simulink model "Problem9_BLDC_Motor"  (R2020b)
settings: Solver=ode45  StartTime=0.0  StopTime=5  MaxStep=0.001  RelTol=1e-5
libraries: fl_lib x23, fl_ps_legacy_lib x15, nesl_utility x7, ee_lib x1
settings Model: Creator=vigne  LastModifiedBy=vigne

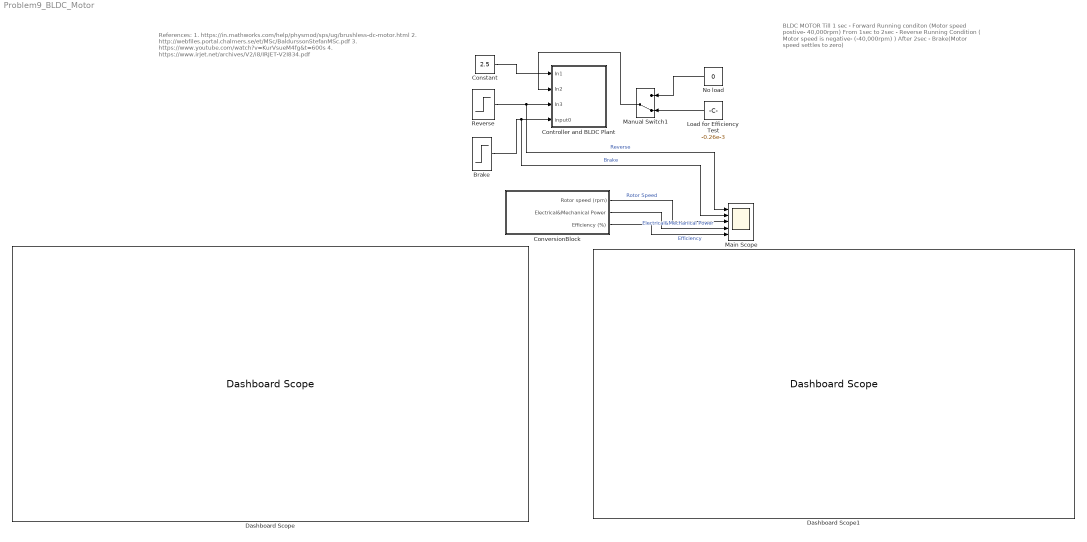
== system Problem9_BLDC_Motor ==
  note: BLDC MOTOR
      |
      | Till 1 sec - Forward Running conditon (Motor speed postive- 40,000rpm)
      |
      | From 1sec to 2sec - Reverse Running Condition ( Motor speed is negative- (-40,000rpm) )
      |
      | After 2sec - Brake(Motor speed settles to zero)
  note: References:
      |
      | 1. https://in.mathworks.com/help/physmod/sps/ug/brushless-dc-motor.html
      | 2. http://webfiles.portal.chalmers.se/et/MSc/BaldurssonStefanMSc.pdf
      | 3. https://www.youtube.com/watch?v=KurVsueM4fg&t=600s
      | 4. https://www.irjet.net/archives/V2/i8/IRJET-V2I834.pdf
  Brake : Step  Time=2  After=5  SampleTime=0
  Constant : Constant  Value=2.5
  Controller and BLDC Plant : Subsystem
  ConversionBlock : Subsystem
  Dashboard Scope : DashboardScope
  Dashboard Scope1 : DashboardScope
  Load for Efficiency Test : Constant  Value=-0.26e-3
  Main Scope : Scope  NumInputPorts=5
  Manual Switch1 : ManualSwitch  CurrentSetting=0
  No load : Constant  Value=0
  Reverse : Step  After=5  SampleTime=0
  wires:
  Load for Efficiency Test/1 -> Manual Switch1/2
  No load/1 -> Manual Switch1/1
  ConversionBlock/1(Rotor speed (rpm)) -> Main Scope/3  "Rotor Speed"
  ConversionBlock/2(Electrical&Mechanical Power) -> Main Scope/4  "Electrical&Mechanical Power"
  ConversionBlock/3(Efficiency (%)) -> Main Scope/5  "Efficiency"
  Constant/1 -> Controller and BLDC Plant/1(In1)
  Manual Switch1/1 -> Controller and BLDC Plant/2(In2)
  Reverse/1 -> Main Scope/1, Controller and BLDC Plant/3(In3)  "Reverse"
  Brake/1 -> Main Scope/2, Controller and BLDC Plant/4(input0)  "Brake"

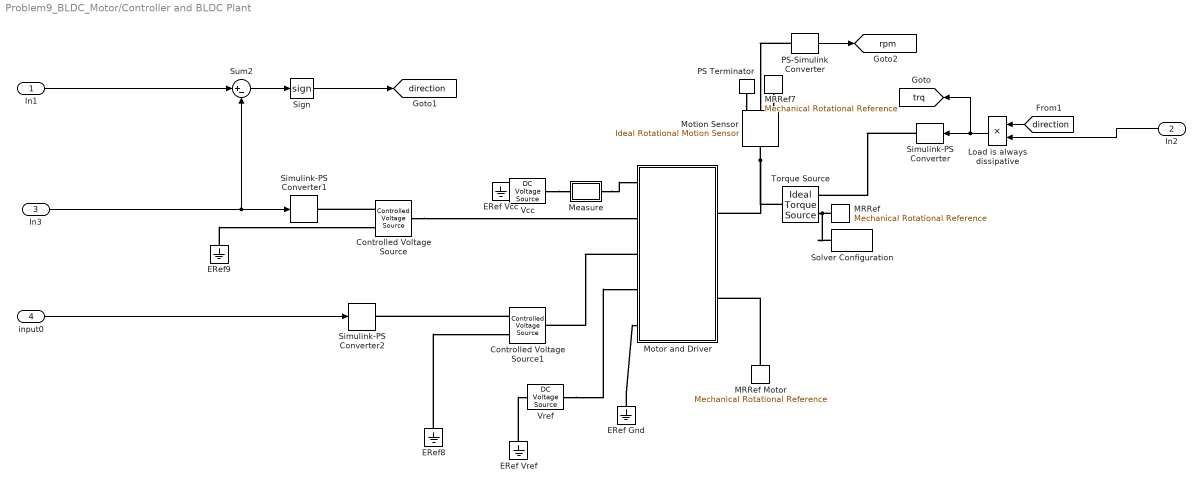
== system Problem9_BLDC_Motor/Controller and BLDC Plant ==
  In1 : Inport
  In2 : Inport  Port=2
  In3 : Inport  Port=3
  input0 : Inport  Port=4
  Controlled Voltage Source : fl_lib/Electrical/Electrical Sources/Controlled Voltage Source
      settings: SourceProductName=Foundation Library
  Controlled Voltage Source1 : fl_lib/Electrical/Electrical Sources/Controlled Voltage Source
      settings: SourceProductName=Foundation Library
  ERef Vcc : fl_lib/Electrical/Electrical Elements/Electrical Reference
      settings: SourceProductName=Foundation Library
  ERef Vref : fl_lib/Electrical/Electrical Elements/Electrical Reference
      settings: SourceProductName=Foundation Library
  ERef Gnd : fl_lib/Electrical/Electrical Elements/Electrical Reference
      settings: SourceProductName=Foundation Library
  ERef8 : fl_lib/Electrical/Electrical Elements/Electrical Reference
      settings: SourceProductName=Foundation Library
  ERef9 : fl_lib/Electrical/Electrical Elements/Electrical Reference
      settings: SourceProductName=Foundation Library
  Load is always dissipative : Product  InputSameDT=on  SaturateOnIntegerOverflow=on  OutDataTypeStr=Inherit: Same as first input
  MRRef : fl_lib/Mechanical/Rotational Elements/Mechanical Rotational Reference
      settings: SourceProductName=Foundation Library
  MRRef Motor : fl_lib/Mechanical/Rotational Elements/Mechanical Rotational Reference
      settings: SourceProductName=Foundation Library
  MRRef7 : fl_lib/Mechanical/Rotational Elements/Mechanical Rotational Reference
      settings: SourceProductName=Foundation Library
  Measure : Subsystem
      mask Display: disp('S');
  Motion Sensor : fl_lib/Mechanical/Mechanical Sensors/Ideal Rotational Motion Sensor  wrap_angle=simscape.enum.onoff.off  offset=0 rad
      settings: SourceProductName=Foundation Library
  Motor and Driver : Subsystem  Tag=PublishSubsystem  mask(Servomotor & Driver){Vcc=12, I0=44e-3, T_i=0.5e-3, eta=41, rpm_eta=40000, trq_eta=0.26e-3, trq_stall=0.44e-3, Kp=0.0000001, Ki=0.000004, Vref_max=5, rpm_max=100000, J=5e-10, rpm0=0}
      mask prompts: Vcc "Nominal voltage (V)"; I0 "No-load DC current to driver (A)"; T_i "Current loop time constant (s)"; eta "Efficiency (%)"; rpm_eta "Speed at which efficiency measured (rpm)"; trq_eta "Torque at which efficiency measured  (Nm)"; trq_stall "Stall torque (Nm)"; Kp "Proportional gain"; Ki "Integral gain"; Vref_max "Maximum reference voltage (V)"; rpm_max "Speed at maximum reference voltage (rpm)"; J "Rotor inerita (kg*m^2)"; rpm0 "Rotor initial speed (rpm)"
      mask help: Implements an abstracted model of a servomotor and driver configured for closed-loop speed control.
      mask DialogControl ParameterTabVar0 Prompt: Electrical
      mask DialogControl ParameterTabVar01 Prompt: Efficiency
      mask DialogControl ParameterTabVar012 Prompt: Mechanical
      mask DialogControl ParameterTabVar0123 Prompt: Controller
  PS Terminator : fl_lib/Physical Signals/Sinks/PS Terminator
      settings: SourceProductName=Foundation Library
  PS-Simulink Converter : nesl_utility/PS-Simulink Converter  PhysicalDomain=network_engine_domain  SubClassName=ps_output  LeftPortType=input  RightPortType=output  PseudoPeriodic=off  Frequencies=[]  Unit=rpm  AffineConversion=off
      settings: SourceProductName=Utilities
  Sign : Signum
  Simulink-PS Converter : nesl_utility/Simulink-PS Converter  PhysicalDomain=network_engine_domain  SubClassName=ps_input  LeftPortType=input  RightPortType=output  PseudoPeriodic=off  Frequencies=[]  NoiseDistribution=none  NoiseParameters=[]  Unit=1  AffineConversion=off  FilteringAndDerivatives=zero  SimscapeFilterOrder=1  InputFilterTimeConstant=.001  UdotUserProvided=0
      settings: SourceProductName=Utilities
  Simulink-PS Converter1 : nesl_utility/Simulink-PS Converter  PhysicalDomain=network_engine_domain  SubClassName=ps_input  LeftPortType=input  RightPortType=output  PseudoPeriodic=off  Frequencies=[]  NoiseDistribution=none  NoiseParameters=[]  Unit=V  AffineConversion=off  FilteringAndDerivatives=zero  SimscapeFilterOrder=1  InputFilterTimeConstant=.001  UdotUserProvided=0
      settings: SourceProductName=Utilities
  Simulink-PS Converter2 : nesl_utility/Simulink-PS Converter  PhysicalDomain=network_engine_domain  SubClassName=ps_input  LeftPortType=input  RightPortType=output  PseudoPeriodic=off  Frequencies=[]  NoiseDistribution=none  NoiseParameters=[]  Unit=V  AffineConversion=off  FilteringAndDerivatives=zero  SimscapeFilterOrder=1  InputFilterTimeConstant=.001  UdotUserProvided=0
      settings: SourceProductName=Utilities
  Solver Configuration : nesl_utility/Solver Configuration  PhysicalDomain=network_engine_domain  SubClassName=solver  LeftPortType=input  RightPortType=generic  Tones=[]  Harmonics=[]  SimulateNoise=off  Profile=off  UseLocalSampling=off  EnableSwitchedLinearOptims=on  FrequencyDomain=off  UseCCode=off  RelTol=0.001  AbsTol=1e-06  MinStep=1e-09  ToWorkspace=off  RevertToSquareIcSolve=off  NumHomotopyIterations=100  PhasorMode=off  PhasorModeNumHarmonics=1  DoDC=off  ResidualTolerance=1e-9  UseLocalSolver=off  LocalSolverChoice=NE_BACKWARD_EULER_ADVANCER  LocalSolverSampleTime=.001  DoFixedCost=off  MaxNonlinIter=3  MaxModeIter=2  ComputeImpulses=off  ImpulseIterations=2  LinearAlgebra=auto  EquationFormulation=NE_TIME_EF  DelaysMemoryBudget=1024  AutomaticFiltering=on  FilteringTimeConstant=0.001  PartitionStorageMethod=AS_NEEDED  PartitionMemoryBudget=1024  PartitionMethod=FAST
      settings: SourceProductName=Utilities
  Sum2 : Sum  Inputs=|+-  InputSameDT=on  SaturateOnIntegerOverflow=on  OutDataTypeStr=Inherit: Same as first input
  Torque Source : fl_lib/Mechanical/Mechanical Sources/Ideal Torque Source
      settings: SourceProductName=Foundation Library
  Vcc : fl_lib/Electrical/Electrical Sources/DC Voltage Source  v0=12 V
      settings: AttributesFormatString=%<v0> %<v0_unit>  SourceProductName=Foundation Library
  Vref : fl_lib/Electrical/Electrical Sources/DC Voltage Source  v0=2 V
      settings: AttributesFormatString=%<v0> %<v0_unit>  SourceProductName=Foundation Library
  tag scope: direction=global, rpm=global, trq=global
  wires:
  Sign/1 -> [direction]
  In1/1 -> Sum2/1
  Load is always dissipative/1 -> [trq], Simulink-PS Converter/1
  [direction] -> Load is always dissipative/1
  PS-Simulink Converter/1 -> [rpm]
  In3/1 -> Simulink-PS Converter1/1, Sum2/2
  Sum2/1 -> Sign/1
  input0/1 -> Simulink-PS Converter2/1
  In2/1 -> Load is always dissipative/2
  connections:
  Motion Sensor/LConn1 -- Motor and Driver/RConn1 -- Torque Source/LConn1
  MRRef/LConn1 -- Solver Configuration/RConn1 -- Torque Source/RConn2
  ERef9/LConn1 -- Controlled Voltage Source/RConn2
  Motor and Driver/LConn3 -- Controlled Voltage Source1/LConn1
  MRRef7/LConn1 -- Motion Sensor/RConn1
  Vcc/LConn1 -- Measure/LConn1
  Simulink-PS Converter/RConn1 -- Torque Source/RConn1
  PS Terminator/LConn1 -- Motion Sensor/RConn3
  MRRef Motor/LConn1 -- Motor and Driver/RConn2
  ERef8/LConn1 -- Controlled Voltage Source1/RConn2
  ERef Gnd/LConn1 -- Motor and Driver/LConn5
  ERef Vcc/LConn1 -- Vcc/RConn1
  PS-Simulink Converter/LConn1 -- Motion Sensor/RConn2
  Controlled Voltage Source/RConn1 -- Simulink-PS Converter1/RConn1
  ERef Vref/LConn1 -- Vref/RConn1
  Vref/LConn1 -- Motor and Driver/LConn4
  Controlled Voltage Source1/RConn1 -- Simulink-PS Converter2/RConn1
  Controlled Voltage Source/LConn1 -- Motor and Driver/LConn2
  Measure/RConn1 -- Motor and Driver/LConn1

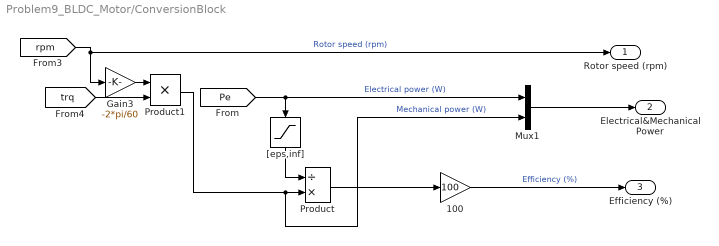
== system Problem9_BLDC_Motor/ConversionBlock ==
  100 : Gain  Gain=100  SaturateOnIntegerOverflow=on  OutDataTypeStr=Inherit: Same as input  ParamDataTypeStr=Inherit: Same as input
  Gain3 : Gain  Gain=-2*pi/60
  Mux1 : Mux  Inputs=2
  Product : Product  Inputs=/*  InputSameDT=on  SaturateOnIntegerOverflow=on  OutDataTypeStr=Inherit: Same as first input
  Product1 : Product
  "[eps,inf]" : Saturate  UpperLimit=inf  LowerLimit=1e-3
  Rotor speed (rpm) : Outport
  Electrical&Mechanical Power : Outport  Port=2
  Efficiency (%) : Outport  Port=3
  wires:
  100/1 -> Efficiency (%)/1  "Efficiency (%)"
  [trq] -> Product1/2
  Product/1 -> 100/1
  [rpm] -> Rotor speed (rpm)/1, Gain3/1  "Rotor speed (rpm)"
  "[eps,inf]"/1 -> Product/1
  [Pe] -> Mux1/1, "[eps,inf]"/1  "Electrical power (W)"
  Mux1/1 -> Electrical&Mechanical Power/1
  Product1/1 -> Mux1/2, Product/2  "Mechanical power (W)"
  Gain3/1 -> Product1/1

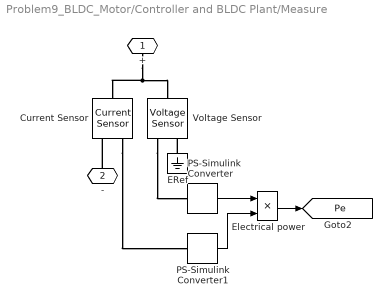
== system Problem9_BLDC_Motor/Controller and BLDC Plant/Measure ==
  Current Sensor : fl_lib/Electrical/Electrical Sensors/Current Sensor
      settings: SourceProductName=Foundation Library
  ERef : fl_lib/Electrical/Electrical Elements/Electrical Reference
      settings: SourceProductName=Foundation Library
  Electrical power : Product  InputSameDT=on  SaturateOnIntegerOverflow=on  OutDataTypeStr=Inherit: Same as first input
  PS-Simulink Converter : nesl_utility/PS-Simulink Converter  PhysicalDomain=network_engine_domain  SubClassName=ps_output  LeftPortType=input  RightPortType=output  PseudoPeriodic=off  Frequencies=[]  Unit=V  AffineConversion=off
      settings: SourceProductName=Utilities
  PS-Simulink Converter1 : nesl_utility/PS-Simulink Converter  PhysicalDomain=network_engine_domain  SubClassName=ps_output  LeftPortType=input  RightPortType=output  PseudoPeriodic=off  Frequencies=[]  Unit=A  AffineConversion=off
      settings: SourceProductName=Utilities
  Voltage Sensor : fl_lib/Electrical/Electrical Sensors/Voltage Sensor
      settings: SourceProductName=Foundation Library
  + : PMIOPort  Side=Left
  - : PMIOPort  Port=2  Side=Right
  tag scope: Pe=global
  wires:
  PS-Simulink Converter/1 -> Electrical power/1
  PS-Simulink Converter1/1 -> Electrical power/2
  Electrical power/1 -> [Pe]
  connections:
  +/RConn1 -- Voltage Sensor/LConn1 -- Current Sensor/LConn1
  Voltage Sensor/RConn1 -- PS-Simulink Converter/LConn1
  ERef/LConn1 -- Voltage Sensor/RConn2
  -/RConn1 -- Current Sensor/RConn2
  Current Sensor/RConn1 -- PS-Simulink Converter1/LConn1

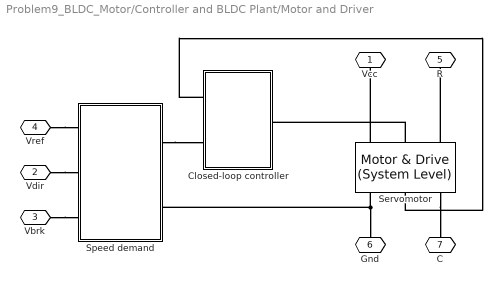
== system Problem9_BLDC_Motor/Controller and BLDC Plant/Motor and Driver ==
  Closed-loop controller : Subsystem
  Servomotor : ee_lib/Electromechanical/Motor & Drive (System Level)  torque_speed_param=1  overtorque_param=ee.enum.electromech.overtorque.no  T_t="[  trq_stall trq_stall trq_stall  0 ] N*m"  T_t_intermittent=[.36, .32, .28, 0] N*m  w_t="[  0 rpm_max 2*rpm_max 2.1*rpm_max ] rpm"  torque_max=0.1 N*m  power_max=30 W  torque_max_intermittent=0.4 N*m  power_max_intermittent=120 W  time_overtorque=30 s  time_recover=60 s  Tc=T_i s  losses_param=1  eff=eta  w_eff=rpm_eta rpm  T_eff=trq_eta N*m  Piron=0 W  Pbase=Vcc*I0 W  w_eff_vec=[-8000 -4000 0 4000 8000] rpm  T_eff_vec=[0 0.03 0.06 0.09] N*m  v_eff_vec=[100, 250, 400] V  losses_mat=[1.49 1.67 2.21 3.10; 0.42 0.69 1.14 2.03; 0.06 0.24 0.78 1.68; 0.42 0.69 1.14 2.03; 1.49 1.67 2.21 3.10] W  efficiency_mat=[95 95 95 95; 95 95 95 95; 95 95 95 95; 95 95 95 95; 95 95 95 95]  losses_mat_3D=ones(5, 4, 3) W  efficiency_mat_3D=95 * ones(5, 4, 3)  Res=0 Ohm  J=J kg*m^2  lam=0 N*m/(rad/s)  speed0=rpm0 rpm  faulted_specify=off  faulted_priority=None  faulted=0  faulted_nominal_specify=off  faulted_nominal_unit=1  faulted_nominal_value=1  torqueLimitContinuous_specify=off  torqueLimitContinuous_priority=None  torqueLimitContinuous=0 N*m  torqueLimitContinuous_nominal_specify=off  torqueLimitContinuous_nominal_unit=N*m  torqueLimitContinuous_nominal_value=1  alpha=3.93e-3 1/K  Tmeas=25 degC  Tmeas2=125 degC  losses_mat_T2=[1.49, 1.74, 2.49, 3.74; .42, .67, 1.42, 2.67; .06, .31, 1.06, 2.31; .42, .67, 1.42, 2.67; 1.49, 1.74, 2.49, 3.74] W  efficiency_mat_T2=[95, 95, 95, 95; 95, 95, 95, 95; 95, 95, 95, 95; 95, 95, 95, 95; 95, 95, 95, 95]  losses_mat_3D_T2=ones(5, 4, 3) W  efficiency_mat_3D_T2=95 * ones(5, 4, 3)  thermal_mass=100 J/K  initial_temperature=25 degC  fault_condition=1  fault_threshold=0.5
      settings: SourceProductName=Electrical
  Speed demand : Subsystem
  Vcc : PMIOPort  Side=Left
  Vdir : PMIOPort  Port=2  Side=Left
  Vbrk : PMIOPort  Port=3  Side=Left
  Vref : PMIOPort  Port=4  Side=Left
  R : PMIOPort  Port=5  Side=Right
  Gnd : PMIOPort  Port=6  Side=Left
  C : PMIOPort  Port=7  Side=Right
  connections:
  Servomotor/LConn2 -- Closed-loop controller/RConn1
  Servomotor/RConn3 -- C/RConn1
  Servomotor/RConn1 -- Gnd/RConn1 -- Speed demand/RConn2
  Vbrk/RConn1 -- Speed demand/LConn3
  Vdir/RConn1 -- Speed demand/LConn2
  Vref/RConn1 -- Speed demand/LConn1
  Servomotor/LConn3 -- R/RConn1
  Servomotor/LConn1 -- Vcc/RConn1
  Closed-loop controller/LConn1 -- Servomotor/RConn2
  Speed demand/RConn1 -- Closed-loop controller/LConn2

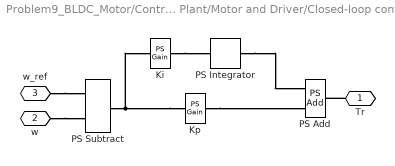
== system Problem9_BLDC_Motor/Controller and BLDC Plant/Motor and Driver/Closed-loop controller ==
  Ki : fl_ps_legacy_lib/Legacy Physical Signals/Functions/PS Gain  gain=Ki
  Kp : fl_ps_legacy_lib/Legacy Physical Signals/Functions/PS Gain  gain=Kp
  PS Add : fl_ps_legacy_lib/Legacy Physical Signals/Functions/PS Add
      settings: SourceProductBaseCode=SS  InternalSimscapePortConfiguration="{\"Bottom\":[],\"Left\":[{\"id\":\"I1\",\"label\":\"\",\"type\":\"input\"},{\"id\":\"I2\",\"label\":\"\",\"type\":\"input\"}],\"Right\":[{\"id\":\"O\",\"label\":\"\",\"type\":\"output\"}],\"Top\":[]}"
  PS Integrator : fl_ps_legacy_lib/Legacy Physical Signals/Linear Operators/PS Integrator  x0=0
      settings: SourceProductBaseCode=SS  InternalSimscapePortConfiguration="{\"Bottom\":[],\"Left\":[{\"id\":\"I\",\"label\":\"\",\"type\":\"input\"}],\"Right\":[{\"id\":\"O\",\"label\":\"\",\"type\":\"output\"}],\"Top\":[]}"
  PS Subtract : fl_ps_legacy_lib/Legacy Physical Signals/Functions/PS Subtract
      settings: SourceProductBaseCode=SS
  Tr : PMIOPort  Side=Right
  w : PMIOPort  Port=2  Side=Left
  w_ref : PMIOPort  Port=3  Side=Left
  connections:
  w/RConn1 -- PS Subtract/LConn2
  w_ref/RConn1 -- PS Subtract/LConn1
  Tr/RConn1 -- PS Add/RConn1
  PS Integrator/RConn1 -- PS Add/LConn1
  Kp/RConn1 -- PS Add/LConn2
  Ki/RConn1 -- PS Integrator/LConn1
  Kp/LConn1 -- PS Subtract/RConn1 -- Ki/LConn1

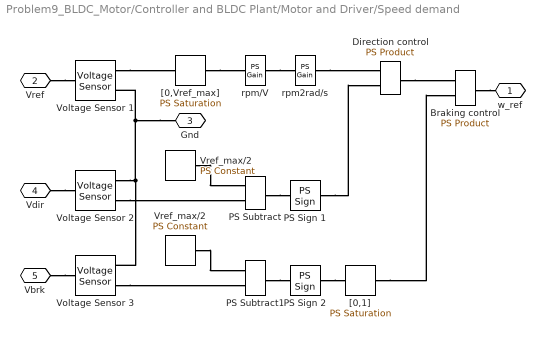
== system Problem9_BLDC_Motor/Controller and BLDC Plant/Motor and Driver/Speed demand ==
  " Vref_max/2 " : fl_lib/Physical Signals/Sources/PS Constant  constant=Vref_max/2
      settings: SourceProductName=Foundation Library
  Braking control : fl_ps_legacy_lib/Legacy Physical Signals/Functions/PS Product
      settings: SourceProductBaseCode=SS
  Direction control : fl_ps_legacy_lib/Legacy Physical Signals/Functions/PS Product
      settings: SourceProductBaseCode=SS
  PS Sign 1 : fl_ps_legacy_lib/Legacy Physical Signals/Nonlinear Operators/PS Sign
      settings: SourceProductBaseCode=SS  InternalSimscapePortConfiguration="{\"Bottom\":[],\"Left\":[{\"id\":\"I\",\"label\":\"\",\"type\":\"input\"}],\"Right\":[{\"id\":\"O\",\"label\":\"\",\"type\":\"output\"}],\"Top\":[]}"
  PS Sign 2 : fl_ps_legacy_lib/Legacy Physical Signals/Nonlinear Operators/PS Sign
      settings: SourceProductBaseCode=SS  InternalSimscapePortConfiguration="{\"Bottom\":[],\"Left\":[{\"id\":\"I\",\"label\":\"\",\"type\":\"input\"}],\"Right\":[{\"id\":\"O\",\"label\":\"\",\"type\":\"output\"}],\"Top\":[]}"
  PS Subtract : fl_ps_legacy_lib/Legacy Physical Signals/Functions/PS Subtract
      settings: SourceProductBaseCode=SS
  PS Subtract1 : fl_ps_legacy_lib/Legacy Physical Signals/Functions/PS Subtract
      settings: SourceProductBaseCode=SS
  Voltage Sensor 1 : fl_lib/Electrical/Electrical Sensors/Voltage Sensor
      settings: SourceProductName=Foundation Library
  Voltage Sensor 2 : fl_lib/Electrical/Electrical Sensors/Voltage Sensor
      settings: SourceProductName=Foundation Library
  Voltage Sensor 3 : fl_lib/Electrical/Electrical Sensors/Voltage Sensor
      settings: SourceProductName=Foundation Library
  Vref_max/2 : fl_lib/Physical Signals/Sources/PS Constant  constant=Vref_max/2
      settings: SourceProductName=Foundation Library
  "[0,1]" : fl_ps_legacy_lib/Legacy Physical Signals/Nonlinear Operators/PS Saturation  upper_limit=5  lower_limit=0
      settings: SourceProductBaseCode=SS  InternalSimscapePortConfiguration="{\"Bottom\":[],\"Left\":[{\"id\":\"I\",\"label\":\"\",\"type\":\"input\"}],\"Right\":[{\"id\":\"O\",\"label\":\"\",\"type\":\"output\"}],\"Top\":[]}"
  "[0,Vref_max]" : fl_ps_legacy_lib/Legacy Physical Signals/Nonlinear Operators/PS Saturation  upper_limit=Vref_max  lower_limit=0
      settings: SourceProductBaseCode=SS  InternalSimscapePortConfiguration="{\"Bottom\":[],\"Left\":[{\"id\":\"I\",\"label\":\"\",\"type\":\"input\"}],\"Right\":[{\"id\":\"O\",\"label\":\"\",\"type\":\"output\"}],\"Top\":[]}"
  rpm/V : fl_ps_legacy_lib/Legacy Physical Signals/Functions/PS Gain  gain=rpm_max/Vref_max
  rpm2rad/s : fl_ps_legacy_lib/Legacy Physical Signals/Functions/PS Gain  gain=2*pi/60
  w_ref : PMIOPort  Side=Right
  Vref : PMIOPort  Port=2  Side=Left
  Gnd : PMIOPort  Port=3  Side=Right
  Vdir : PMIOPort  Port=4  Side=Left
  Vbrk : PMIOPort  Port=5  Side=Left
  connections:
  "[0,1]"/RConn1 -- Braking control/LConn2
  Braking control/RConn1 -- w_ref/RConn1
  Direction control/RConn1 -- Braking control/LConn1
  PS Sign 2/RConn1 -- "[0,1]"/LConn1
  PS Subtract1/RConn1 -- PS Sign 2/LConn1
  " Vref_max/2 "/RConn1 -- PS Subtract1/LConn1
  Voltage Sensor 3/RConn1 -- PS Subtract1/LConn2
  Vbrk/RConn1 -- Voltage Sensor 3/LConn1
  Vref_max/2/RConn1 -- PS Subtract/LConn1
  Voltage Sensor 2/RConn1 -- PS Subtract/LConn2
  PS Sign 1/RConn1 -- Direction control/LConn2
  rpm2rad/s/RConn1 -- Direction control/LConn1
  PS Subtract/RConn1 -- PS Sign 1/LConn1
  Vdir/RConn1 -- Voltage Sensor 2/LConn1
  Gnd/RConn1 -- Voltage Sensor 3/RConn2 -- Voltage Sensor 2/RConn2 -- Voltage Sensor 1/RConn2
  Vref/RConn1 -- Voltage Sensor 1/LConn1
  rpm/V/RConn1 -- rpm2rad/s/LConn1
  "[0,Vref_max]"/RConn1 -- rpm/V/LConn1
  Voltage Sensor 1/RConn1 -- "[0,Vref_max]"/LConn1
